simulink model "tuningPIDUpgraded"  (R2017a)
settings: Solver=VariableStepAuto  StartTime=0.0  StopTime=2000.0  RelTol=1e-3
values from neighbouring files (symbols this model uses):
  G1 = tf(num,den,'InputDelay',[0,tau_C,0,0],'OutputDelay',[tau,0])    [TAP_Projekt1.m]    (also in decoupling.m = collect(G1); testWithDecouplers.m = collect(G1))
libraries: cstblocks x8, simulink x2
settings Model: Creator=Barteux  LastModifiedBy=Barteux

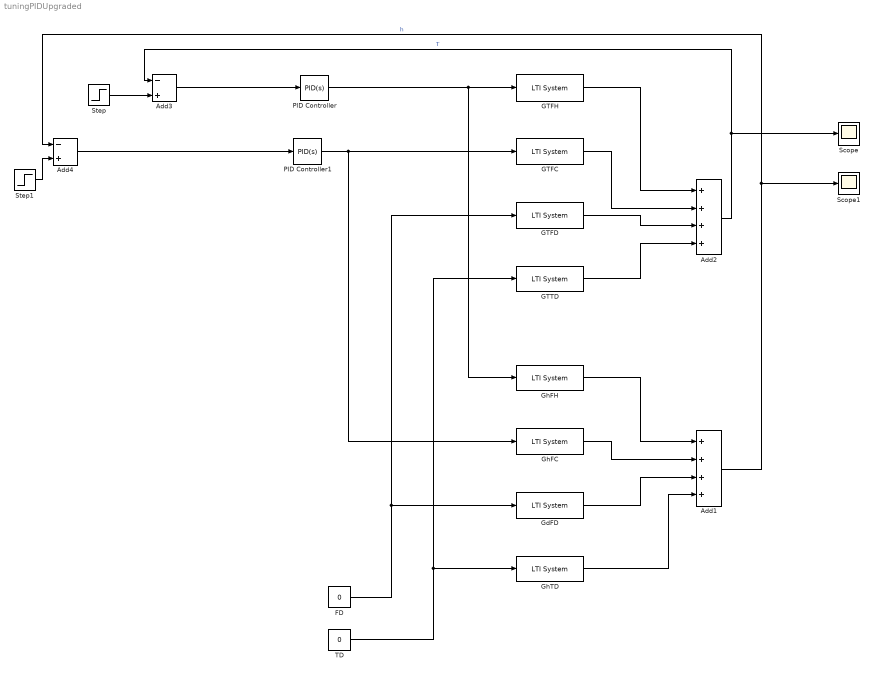
== system tuningPIDUpgraded ==
  Add1 : Sum  Inputs=++++
  Add2 : Sum  Inputs=++++
  Add3 : Sum  Inputs=-+
  Add4 : Sum  Inputs=-+
  FD : Constant  Value=0
  GTFC : cstblocks/LTI System  sys=G1(1,2)  IC=[]
  GTFD : cstblocks/LTI System  sys=G1(1,3)  IC=[]
  GTFH : cstblocks/LTI System  sys=G1(1,1)  IC=[]
  GTTD : cstblocks/LTI System  sys=G1(1,4)  IC=[]
  GdFD : cstblocks/LTI System  sys=G1(2,3)  IC=[]
  GhFC : cstblocks/LTI System  sys=G1(2,2)  IC=[]
  GhFH : cstblocks/LTI System  sys=G1(2,1)  IC=[]
  GhTD : cstblocks/LTI System  sys=G1(2,4)  IC=[]
  PID Controller : simulink/Continuous/PID Controller  Controller=PID  TimeDomain=Continuous-time  SampleTime=-1  IntegratorMethod=Forward Euler  FilterMethod=Forward Euler  Form=Parallel  UseFilter=on  ControllerParametersSource=internal  P=0.528829547017946  I=0.024693739630127  D=0  N=100  InitialConditionSource=internal  InitialConditionForIntegrator=0  InitialConditionForFilter=0  ExternalReset=none  LimitOutput=off  UpperSaturationLimit=inf  LowerSaturationLimit=-inf  LinearizeAsGain=on  AntiWindupMode=none  Kb=1  TrackingMode=off  Kt=1  PParamMin=[]  PParamMax=[]  IParamMin=[]  IParamMax=[]  DParamMin=[]  DParamMax=[]  NParamMin=[]  NParamMax=[]  KbParamMin=[]  KbParamMax=[]  KtParamMin=[]  KtParamMax=[]  POutMin=[]  POutMax=[]  IOutMin=[]  IOutMax=[]  DOutMin=[]  DOutMax=[]  NOutMin=[]  NOutMax=[]  KbOutMin=[]  KbOutMax=[]  KtOutMin=[]  KtOutMax=[]  IntegratorOutMin=[]  IntegratorOutMax=[]  FilterOutMin=[]  FilterOutMax=[]  SumOutMin=[]  SumOutMax=[]  SumI1OutMin=[]  SumI1OutMax=[]  SumI2OutMin=[]  SumI2OutMax=[]  SumI3OutMin=[]  SumI3OutMax=[]  SumDOutMin=[]  SumDOutMax=[]  SaturationOutMin=[]  SaturationOutMax=[]  IntegratorContinuousStateAttributes=''  IntegratorStateMustResolveToSignalObject=off  IntegratorRTWStateStorageClass=Auto  FilterContinuousStateAttributes=''  FilterStateMustResolveToSignalObject=off  FilterRTWStateStorageClass=Auto  DifferentiatorICPrevScaledInput=0  DifferentiatorOutMin=[]  DifferentiatorOutMax=[]  InitialConditionSetting=State (most efficient)
  PID Controller1 : simulink/Continuous/PID Controller  Controller=PID  TimeDomain=Continuous-time  SampleTime=-1  IntegratorMethod=Forward Euler  FilterMethod=Forward Euler  Form=Parallel  UseFilter=on  ControllerParametersSource=internal  P=0.216337475454881  I=0.00240325675501345  D=0  N=100  InitialConditionSource=internal  InitialConditionForIntegrator=0  InitialConditionForFilter=0  ExternalReset=none  LimitOutput=off  UpperSaturationLimit=inf  LowerSaturationLimit=-inf  LinearizeAsGain=on  AntiWindupMode=none  Kb=1  TrackingMode=off  Kt=1  PParamMin=[]  PParamMax=[]  IParamMin=[]  IParamMax=[]  DParamMin=[]  DParamMax=[]  NParamMin=[]  NParamMax=[]  KbParamMin=[]  KbParamMax=[]  KtParamMin=[]  KtParamMax=[]  POutMin=[]  POutMax=[]  IOutMin=[]  IOutMax=[]  DOutMin=[]  DOutMax=[]  NOutMin=[]  NOutMax=[]  KbOutMin=[]  KbOutMax=[]  KtOutMin=[]  KtOutMax=[]  IntegratorOutMin=[]  IntegratorOutMax=[]  FilterOutMin=[]  FilterOutMax=[]  SumOutMin=[]  SumOutMax=[]  SumI1OutMin=[]  SumI1OutMax=[]  SumI2OutMin=[]  SumI2OutMax=[]  SumI3OutMin=[]  SumI3OutMax=[]  SumDOutMin=[]  SumDOutMax=[]  SaturationOutMin=[]  SaturationOutMax=[]  IntegratorContinuousStateAttributes=''  IntegratorStateMustResolveToSignalObject=off  IntegratorRTWStateStorageClass=Auto  FilterContinuousStateAttributes=''  FilterStateMustResolveToSignalObject=off  FilterRTWStateStorageClass=Auto  DifferentiatorICPrevScaledInput=0  DifferentiatorOutMin=[]  DifferentiatorOutMax=[]  InitialConditionSetting=State (most efficient)
  Scope : Scope
  Scope1 : Scope
  Step : Step  SampleTime=0
  Step1 : Step  SampleTime=0
  TD : Constant  Value=0
  wires:
  TD/1 -> GTTD/1, GhTD/1
  FD/1 -> GdFD/1, GTFD/1
  GhFH/1 -> Add1/1
  GhFC/1 -> Add1/2
  GdFD/1 -> Add1/3
  GhTD/1 -> Add1/4
  GTFH/1 -> Add2/1
  GTFC/1 -> Add2/2
  GTFD/1 -> Add2/3
  GTTD/1 -> Add2/4
  Add2/1 -> Add3/1, Scope/1  "T"
  Add1/1 -> Add4/1, Scope1/1  "h"
  Add3/1 -> PID Controller/1
  Step/1 -> Add3/2
  Add4/1 -> PID Controller1/1
  Step1/1 -> Add4/2
  PID Controller1/1 -> GhFC/1, GTFC/1
  PID Controller/1 -> GhFH/1, GTFH/1
